simulink model "Z2"  (R2015b)
settings: Solver=FixedStepAuto  StartTime=0.0  StopTime=5.0  FixedStep=1e-4  RelTol=1e-3
undefined symbols (not defined in the file): T
settings Model: Creator=Erdal  LastModifiedBy=Erdal

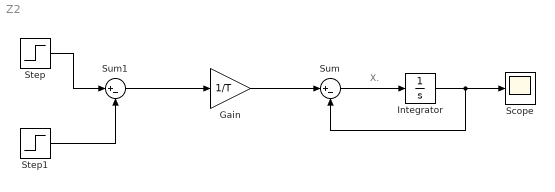
== system Z2 ==
  note: X.
  Gain : Gain  Gain=1/T
  Integrator : Integrator  InitialCondition=5
  Scope : Scope
  Step : Step  Time=0  SampleTime=0
  Step1 : Step  Time=T  SampleTime=0
  Sum : Sum  Inputs=|+-
  Sum1 : Sum  Inputs=|+-
  wires:
  Step1/1 -> Sum1/2
  Step/1 -> Sum1/1
  Sum1/1 -> Gain/1
  Gain/1 -> Sum/1
  Sum/1 -> Integrator/1
  Integrator/1 -> Sum/2, Scope/1
